simulink model "SEMINAR_DFIG_withsubsys"  (R2014a)
settings: Solver=ode23tb  StartTime=0.0  StopTime=1  FixedStep=1e-9  RelTol=1e-8  AbsTol=1e-8
libraries: powerlib x18, powerlib_meascontrol x13, simulink x7
settings Model: BufferReuse=off  Creator=user  LastModifiedBy=ninad gaikawad
settings SolverCC: MaxConsecutiveZCs=1000000  MaxConsecutiveMinStep=1000000  ZeroCrossAlgorithm=Adaptive  SolverResetMethod=Robust
settings OptimizationCC: BlockReduction=off  OptimizeBlockIOStorage=off  BufferReuse=off  GlobalBufferReuse=off  ExpressionFolding=off  LocalBlockOutputs=off

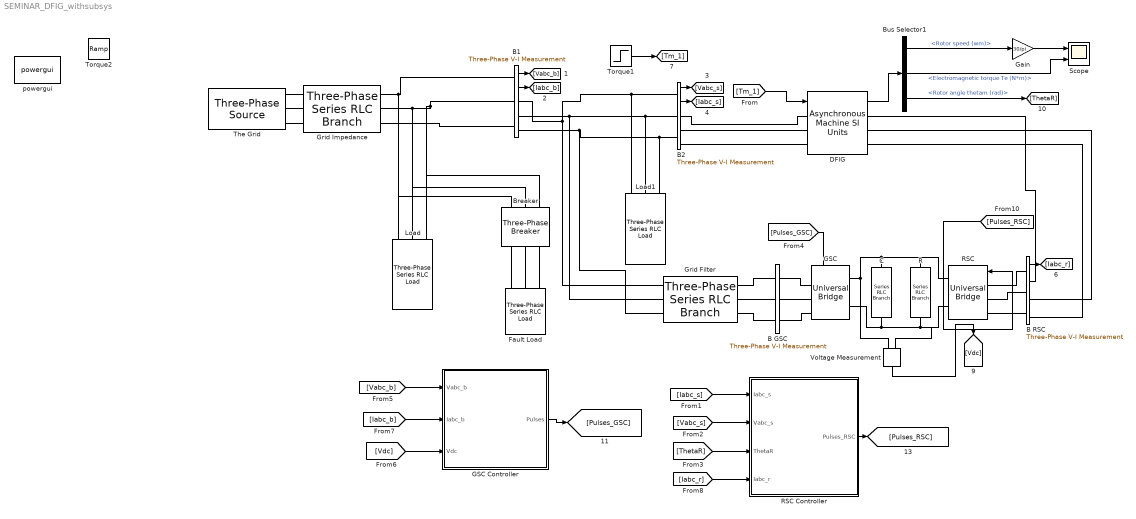
== system SEMINAR_DFIG_withsubsys ==
  B GSC : powerlib/Measurements/Three-Phase V-I Measurement  VoltageMeasurement=no  SetLabelV=off  LabelV=Vabc  Vpu=off  VpuLL=off  CurrentMeasurement=no  SetLabelI=off  LabelI=Iabc  Ipu=off  Pbase=100e6  Vbase=500e3  OutputType=Complex  PhasorSimulation=off  PSBequivalent=0
  B RSC : powerlib/Measurements/Three-Phase V-I Measurement  VoltageMeasurement=no  SetLabelV=off  LabelV=Vabc  Vpu=off  VpuLL=off  CurrentMeasurement=yes  SetLabelI=off  LabelI=Iabc  Ipu=off  Pbase=100e6  Vbase=500e3  OutputType=Complex  PhasorSimulation=off  PSBequivalent=0
  B1 : powerlib/Measurements/Three-Phase V-I Measurement  VoltageMeasurement=phase-to-ground  SetLabelV=off  LabelV=Vabc  Vpu=off  VpuLL=off  CurrentMeasurement=yes  SetLabelI=off  LabelI=Iabc  Ipu=off  Pbase=100e6  Vbase=500e3  OutputType=Complex  PhasorSimulation=off  PSBequivalent=0
  B2 : powerlib/Measurements/Three-Phase V-I Measurement  VoltageMeasurement=phase-to-ground  SetLabelV=off  LabelV=Vabc  Vpu=off  VpuLL=off  CurrentMeasurement=yes  SetLabelI=off  LabelI=Iabc  Ipu=off  Pbase=100e6  Vbase=500e3  OutputType=Complex  PhasorSimulation=off  PSBequivalent=0
  Breaker : powerlib/Elements/Three-Phase Breaker  InitialState=open  SwitchA=on  SwitchB=on  SwitchC=on  SwitchTimes="[1/60  5/60]"  External=off  BreakerResistance=0.01  SnubberResistance=1e6  SnubberCapacitance=inf  Measurements=None
  Bus Selector1 : BusSelector  OutputSignals=Mechanical.Rotor speed (wm),Mechanical.Electromagnetic torque Te (N*m),Mechanical.Rotor angle thetam (rad)
  C : powerlib/Elements/Series RLC Branch  LConnTagsString=__new0  RConnTagsString=__new0  BranchType=C  Resistance=1  Inductance=1e-3  SetiL0=off  InitialCurrent=0  Capacitance=0.0024  Setx0=off  InitialVoltage=0  Measurements=None
  DFIG : powerlib/Machines/Asynchronous Machine SI Units  PresetModel=No  MechanicalLoad=Torque Tm  ShowDetailedParameters=on  RotorType=Wound  ReferenceFrame=Rotor  Units=SI  MeasurementBus=off  NominalParameters=[7.5e3 415 50]  Stator=[1.06 0.2065]  Rotor=[0.80 0.0810]  Cage1=[ 0.022 0.226/377]  Cage2=[ 0.022 0.226/377]  Lm=0.02135  Mechanical=[0.03 0.02187 3]  PolePairs=2  InitialConditions=[1 0 0 0 0 0 0 0]  SimulateSaturation=off  Saturation=[14.03593122, 27.81365428, 53.79336849, 72.68890987, 97.98006896, 148.6815601, 215.7428561, 302.9841135, 420.4778367 ; 230, 322, 414, 460, 506, 552, 598, 644, 690]  LoadFlowParameters=1492000  TsPowergui=0  TsBlock=-1  IterativeModel=Trapezoidal non iterative  Pmec=0
  Fault Load : powerlib/Elements/Three-Phase Series RLC Load  LConnTagsString=A|B|C  Configuration=Y (grounded)  NominalVoltage=1000  NominalFrequency=60  ActivePower=0.05e+3  InductivePower=0  CapacitivePower=0  Measurements=None  LoadType=constant Z
  GSC : powerlib/Power Electronics/Universal Bridge  Arms=3  SnubberResistance=1e5  SnubberCapacitance=inf  Device=IGBT / Diodes  Ron=1e-3  Lon=0  ForwardVoltages="[  0  0  ]"  ForwardVoltage=0  GTOparameters=[ 10e-6 , 20e-6 ]  IGBTparameters=[ 1e-6 , 2e-6 ]  Measurements=None  Measurements_2=None  converterType=Rectifier
  GSC Controller : Subsystem
  Gain : Gain  Gain=30/pi
  Grid Filter : powerlib/Elements/Three-Phase Series RLC Branch  LConnTagsString=A|B|C  RConnTagsString=A|B|C  BranchType=RL  Resistance=0.1  Inductance=0.012  Capacitance=1e-6  Measurements=None
  Grid Impedance : powerlib/Elements/Three-Phase Series RLC Branch  LConnTagsString=A|B|C  RConnTagsString=A|B|C  BranchType=RL  Resistance=1  Inductance=1e-3  Capacitance=1e-6  Measurements=None
  Load : powerlib/Elements/Three-Phase Series RLC Load  LConnTagsString=A|B|C  Configuration=Y (grounded)  NominalVoltage=1000  NominalFrequency=50  ActivePower=5e+3  InductivePower=0  CapacitivePower=0  Measurements=None  LoadType=constant Z
  Load1 : powerlib/Elements/Three-Phase Series RLC Load  LConnTagsString=A|B|C  Configuration=Y (grounded)  NominalVoltage=1000  NominalFrequency=50  ActivePower=5e+4  InductivePower=0  CapacitivePower=0  Measurements=None  LoadType=constant Z
  R : powerlib/Elements/Series RLC Branch  LConnTagsString=__new0  RConnTagsString=__new0  BranchType=R  Resistance=1  Inductance=1e-3  SetiL0=off  InitialCurrent=0  Capacitance=1e-6  Setx0=off  InitialVoltage=0  Measurements=None
  RSC : powerlib/Power Electronics/Universal Bridge  Arms=3  SnubberResistance=1e5  SnubberCapacitance=inf  Device=IGBT / Diodes  Ron=1e-3  Lon=0  ForwardVoltages="[  0  0  ]"  ForwardVoltage=0  GTOparameters=[ 10e-6 , 20e-6 ]  IGBTparameters=[ 1e-6 , 2e-6 ]  Measurements=None  Measurements_2=None  converterType=Rectifier
  RSC Controller : Subsystem
  Scope : Scope  NumInputPorts=2
      settings: YMin=-5~-5  YMax=5~5
  The Grid : powerlib/Electrical Sources/Three-Phase Source  Voltage=415  PhaseAngle=0  Frequency=50  InternalConnection=Yg  SpecifyImpedance=off  Resistance=0.8929  Inductance=0  ShortCircuitLevel=100e6  BaseVoltage=25e3  XRratio=7  BusType=swing  Pref=0  Qref=0  Qmin=-inf  Qmax=inf
  Torque1 : Step  Time=0.5  After=-25  SampleTime=0
  Torque2 : simulink/Sources/Ramp  slope=-1  start=0  X0=0
  Voltage Measurement : powerlib/Measurements/Voltage Measurement  PhasorSimulation=off  OutputType=Complex  PSBequivalent=0
  powergui : powerlib/powergui  Priority=1  SimulationMode=Continuous  SolverType=Tustin  SampleTime=50e-6  frequency=60  SPID=off  DisableSnubberDevices=off  DisableRonSwitches=off  DisableVfSwitches=off  SwTol=0  Interpol=off  DisplayEquations=off  Ts=0  methode=off  frequencyindice=50  Pbase=100e6  ErrMax=1e-4  Iterations=50  UnitsV=kV  UnitsW=MW  FunctionMessages=off  echomessages=off  HookPort=off  EnableUseOfTLC=off  x0status=blocks  RestoreLinks=warning  ResistiveCurrentMeasurement=off  Frange=[0:2:500]  Ylog=off  Xlog=on  ShowGrid=off  save=off  variable=ZData  structure=0  ZoomFFT=off  StartTime=0.0  cycles=1  DisplayStyle=1  fundamental=60  FreqAxis=off  MaxFrequency=1000  frequencyindicesteady=1  RmsSteady=1  display=off
  wires:
  DFIG/1 -> Bus Selector1/1
  B1/1 -> [Vabc_b]
  B1/2 -> [Iabc_b]
  B2/1 -> [Vabc_s]
  B2/2 -> [Iabc_s]
  B RSC/1 -> [Iabc_r]
  Torque1/1 -> [Tm_1]
  [Tm_1] -> DFIG/1
  Voltage Measurement/1 -> [Vdc]
  [Pulses_GSC] -> GSC/1
  [Vabc_b] -> GSC Controller/1(Vabc_b)
  [Vdc] -> GSC Controller/3(Vdc)
  GSC Controller/1(Pulses) -> [Pulses_GSC]
  [Iabc_b] -> GSC Controller/2(Iabc_b)
  Bus Selector1/1 -> Gain/1  "<Rotor speed (wm)>"
  Gain/1 -> Scope/1
  Bus Selector1/3 -> [ThetaR]  "<Rotor angle thetam (rad)>"
  Bus Selector1/2 -> Scope/2  "<Electromagnetic torque Te (N*m)>"
  [Iabc_s] -> RSC Controller/1(Iabc_s)
  [ThetaR] -> RSC Controller/3(ThetaR)
  [Iabc_r] -> RSC Controller/4(Iabc_r)
  RSC Controller/1(Pulses_RSC) -> [Pulses_RSC]
  [Vabc_s] -> RSC Controller/2(Vabc_s)
  [Pulses_RSC] -> RSC/1
  connections:
  GSC/RConn1 -- RSC/RConn1 -- R/LConn1 -- C/LConn1 -- Voltage Measurement/LConn1
  GSC/RConn2 -- Voltage Measurement/LConn2 -- RSC/RConn2 -- R/RConn1 -- C/RConn1
  The Grid/RConn1 -- Grid Impedance/LConn1
  The Grid/RConn2 -- Grid Impedance/LConn2
  The Grid/RConn3 -- Grid Impedance/LConn3
  Breaker/RConn1 -- Fault Load/LConn1
  Breaker/RConn2 -- Fault Load/LConn2
  Grid Impedance/RConn2 -- Breaker/LConn2 -- Load/LConn2 -- Breaker/LConn3 -- Load/LConn3 -- B1/LConn2
  Grid Impedance/RConn3 -- B1/LConn3
  B1/RConn2 -- Grid Filter/LConn2 -- Load1/LConn2 -- B2/LConn2
  B1/RConn3 -- Grid Filter/LConn3 -- Load1/LConn3 -- B2/LConn3
  B2/LConn1 -- Load1/LConn1 -- Grid Filter/LConn1 -- B1/RConn1
  Grid Impedance/RConn1 -- Breaker/LConn1 -- Load/LConn1 -- B1/LConn1
  Fault Load/LConn3 -- Breaker/RConn3
  B2/RConn1 -- DFIG/LConn1
  B2/RConn2 -- DFIG/LConn2
  B2/RConn3 -- DFIG/LConn3
  Grid Filter/RConn1 -- B GSC/LConn1
  Grid Filter/RConn2 -- B GSC/LConn2
  Grid Filter/RConn3 -- B GSC/LConn3
  B GSC/RConn3 -- GSC/LConn3
  B GSC/RConn2 -- GSC/LConn2
  B GSC/RConn1 -- GSC/LConn1
  RSC/LConn1 -- B RSC/LConn1
  RSC/LConn2 -- B RSC/LConn2
  RSC/LConn3 -- B RSC/LConn3
  DFIG/RConn1 -- B RSC/RConn1
  DFIG/RConn2 -- B RSC/RConn2
  DFIG/RConn3 -- B RSC/RConn3

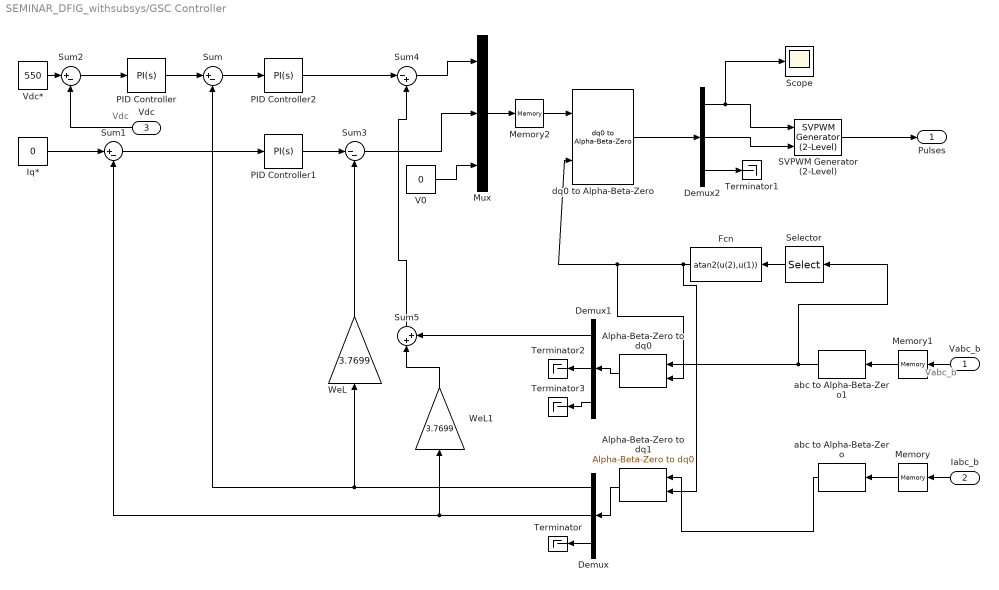
== system SEMINAR_DFIG_withsubsys/GSC Controller ==
  note: Vdc
  note: Vabc_b
  Vabc_b : Inport
  Iabc_b : Inport  Port=2
  Vdc : Inport  Port=3
  Alpha-Beta-Zero to dq0 : powerlib_meascontrol/Transformations/Alpha-Beta-Zero to dq0  Alignment=Aligned with phase A axis
  Alpha-Beta-Zero to dq1 : powerlib_meascontrol/Transformations/Alpha-Beta-Zero to dq0  Alignment=Aligned with phase A axis
  Demux : Demux  Outputs=3
  Demux1 : Demux  Outputs=3
  Demux2 : Demux  Outputs=3
  Fcn : Fcn  Expr=atan2(u(2),u(1))
  Iq* : Constant  Value=0
  Memory : Memory  X0=1
  Memory1 : Memory  X0=100
  Memory2 : Memory  X0=1
  Mux : Mux  Inputs=3
  PID Controller : simulink/Continuous/PID Controller  Controller=PI  TimeDomain=Continuous-time  SampleTime=1  IntegratorMethod=Forward Euler  FilterMethod=Forward Euler  Form=Parallel  P=0.028073571427237  I=0.0618958834223804  D=0  N=100  InitialConditionSource=internal  InitialConditionForIntegrator=0  InitialConditionForFilter=0  ExternalReset=none  LimitOutput=off  UpperSaturationLimit=1  LowerSaturationLimit=-1  LinearizeAsGain=on  AntiWindupMode=none  Kb=1  TrackingMode=off  Kt=1  PParamMin=[]  PParamMax=[]  IParamMin=[]  IParamMax=[]  DParamMin=[]  DParamMax=[]  NParamMin=[]  NParamMax=[]  KbParamMin=[]  KbParamMax=[]  KtParamMin=[]  KtParamMax=[]  POutMin=[]  POutMax=[]  IOutMin=[]  IOutMax=[]  DOutMin=[]  DOutMax=[]  NOutMin=[]  NOutMax=[]  KbOutMin=[]  KbOutMax=[]  KtOutMin=[]  KtOutMax=[]  IntegratorOutMin=[]  IntegratorOutMax=[]  FilterOutMin=[]  FilterOutMax=[]  SumOutMin=[]  SumOutMax=[]  SumI1OutMin=[]  SumI1OutMax=[]  SumI2OutMin=[]  SumI2OutMax=[]  SumI3OutMin=[]  SumI3OutMax=[]  SumDOutMin=[]  SumDOutMax=[]  SaturationOutMin=[]  SaturationOutMax=[]  IntegratorContinuousStateAttributes=''  IntegratorStateMustResolveToSignalObject=off  IntegratorRTWStateStorageClass=Auto  FilterContinuousStateAttributes=''  FilterStateMustResolveToSignalObject=off  FilterRTWStateStorageClass=Auto
  PID Controller1 : simulink/Continuous/PID Controller  Controller=PI  TimeDomain=Continuous-time  SampleTime=1  IntegratorMethod=Forward Euler  FilterMethod=Forward Euler  Form=Parallel  P=8.37826727980584  I=0.0516922409916327  D=0  N=100  InitialConditionSource=internal  InitialConditionForIntegrator=0  InitialConditionForFilter=0  ExternalReset=none  LimitOutput=off  UpperSaturationLimit=1  LowerSaturationLimit=-1  LinearizeAsGain=on  AntiWindupMode=none  Kb=1  TrackingMode=off  Kt=1  PParamMin=[]  PParamMax=[]  IParamMin=[]  IParamMax=[]  DParamMin=[]  DParamMax=[]  NParamMin=[]  NParamMax=[]  KbParamMin=[]  KbParamMax=[]  KtParamMin=[]  KtParamMax=[]  POutMin=[]  POutMax=[]  IOutMin=[]  IOutMax=[]  DOutMin=[]  DOutMax=[]  NOutMin=[]  NOutMax=[]  KbOutMin=[]  KbOutMax=[]  KtOutMin=[]  KtOutMax=[]  IntegratorOutMin=[]  IntegratorOutMax=[]  FilterOutMin=[]  FilterOutMax=[]  SumOutMin=[]  SumOutMax=[]  SumI1OutMin=[]  SumI1OutMax=[]  SumI2OutMin=[]  SumI2OutMax=[]  SumI3OutMin=[]  SumI3OutMax=[]  SumDOutMin=[]  SumDOutMax=[]  SaturationOutMin=[]  SaturationOutMax=[]  IntegratorContinuousStateAttributes=''  IntegratorStateMustResolveToSignalObject=off  IntegratorRTWStateStorageClass=Auto  FilterContinuousStateAttributes=''  FilterStateMustResolveToSignalObject=off  FilterRTWStateStorageClass=Auto
  PID Controller2 : simulink/Continuous/PID Controller  Controller=PI  TimeDomain=Continuous-time  SampleTime=1  IntegratorMethod=Forward Euler  FilterMethod=Forward Euler  Form=Parallel  P=8.37826727980584  I=0.0516922409916327  D=0  N=100  InitialConditionSource=internal  InitialConditionForIntegrator=0  InitialConditionForFilter=0  ExternalReset=none  LimitOutput=off  UpperSaturationLimit=1  LowerSaturationLimit=-1  LinearizeAsGain=on  AntiWindupMode=none  Kb=1  TrackingMode=off  Kt=1  PParamMin=[]  PParamMax=[]  IParamMin=[]  IParamMax=[]  DParamMin=[]  DParamMax=[]  NParamMin=[]  NParamMax=[]  KbParamMin=[]  KbParamMax=[]  KtParamMin=[]  KtParamMax=[]  POutMin=[]  POutMax=[]  IOutMin=[]  IOutMax=[]  DOutMin=[]  DOutMax=[]  NOutMin=[]  NOutMax=[]  KbOutMin=[]  KbOutMax=[]  KtOutMin=[]  KtOutMax=[]  IntegratorOutMin=[]  IntegratorOutMax=[]  FilterOutMin=[]  FilterOutMax=[]  SumOutMin=[]  SumOutMax=[]  SumI1OutMin=[]  SumI1OutMax=[]  SumI2OutMin=[]  SumI2OutMax=[]  SumI3OutMin=[]  SumI3OutMax=[]  SumDOutMin=[]  SumDOutMax=[]  SaturationOutMin=[]  SaturationOutMax=[]  IntegratorContinuousStateAttributes=''  IntegratorStateMustResolveToSignalObject=off  IntegratorRTWStateStorageClass=Auto  FilterContinuousStateAttributes=''  FilterStateMustResolveToSignalObject=off  FilterRTWStateStorageClass=Auto
  SVPWM Generator (2-Level) : powerlib_meascontrol/Pulse & Signal Generators/SVPWM Generator (2-Level)  InputType=alpha-beta components  SwitchingPattern=Pattern #1  Fc=27*50  ParUref=[0.8 -30 50]  Ts=0
  Scope : Scope
  Selector : Selector  InputPortWidth=3  Indices=[1 2]
  Sum : Sum  Inputs=|+-
  Sum1 : Sum  Inputs=|+-
  Sum2 : Sum  Inputs=|+-
  Sum3 : Sum  Inputs=|--
  Sum4 : Sum  Inputs=|-+
  Sum5 : Sum  Inputs=|++
  Terminator{,1..3} (4 alike) : Terminator
  V0 : Constant  Value=0
  Vdc* : Constant  Value=550
  WeL : Gain  Gain=3.7699
  WeL1 : Gain  Gain=3.7699
  abc to Alpha-Beta-Zero : powerlib_meascontrol/Transformations/abc to Alpha-Beta-Zero
  abc to Alpha-Beta-Zero1 : powerlib_meascontrol/Transformations/abc to Alpha-Beta-Zero
  dq0 to Alpha-Beta-Zero : powerlib_meascontrol/Transformations/dq0 to Alpha-Beta-Zero  Alignment=90 degrees behind phase A axis
  Pulses : Outport
  wires:
  Demux1/3 -> Terminator3/1
  Demux/3 -> Terminator/1
  Alpha-Beta-Zero to dq1/1 -> Demux/1
  Fcn/1 -> Alpha-Beta-Zero to dq1/2, dq0 to Alpha-Beta-Zero/2, Alpha-Beta-Zero to dq0/2
  abc to Alpha-Beta-Zero1/1 -> Selector/1, Alpha-Beta-Zero to dq0/1
  abc to Alpha-Beta-Zero/1 -> Alpha-Beta-Zero to dq1/1
  Alpha-Beta-Zero to dq0/1 -> Demux1/1
  Vabc_b/1 -> Memory1/1
  Demux1/2 -> Terminator2/1
  Iabc_b/1 -> Memory/1
  Selector/1 -> Fcn/1
  Demux2/3 -> Terminator1/1
  Demux2/2 -> SVPWM Generator (2-Level)/2
  Demux2/1 -> Scope/1, SVPWM Generator (2-Level)/1
  dq0 to Alpha-Beta-Zero/1 -> Demux2/1
  SVPWM Generator (2-Level)/1 -> Pulses/1
  Mux/1 -> Memory2/1
  Sum4/1 -> Mux/1
  PID Controller1/1 -> Sum3/1
  Demux/1 -> Sum/2, WeL/1
  Demux1/1 -> Sum5/2
  PID Controller2/1 -> Sum4/1
  Demux/2 -> Sum1/2, WeL1/1
  Sum1/1 -> PID Controller1/1
  Sum5/1 -> Sum4/2
  Sum3/1 -> Mux/2
  WeL1/1 -> Sum5/1
  PID Controller/1 -> Sum/1
  Iq*/1 -> Sum1/1
  WeL/1 -> Sum3/2
  Sum2/1 -> PID Controller/1
  Vdc*/1 -> Sum2/1
  V0/1 -> Mux/3
  Sum/1 -> PID Controller2/1
  Vdc/1 -> Sum2/2
  Memory1/1 -> abc to Alpha-Beta-Zero1/1
  Memory/1 -> abc to Alpha-Beta-Zero/1
  Memory2/1 -> dq0 to Alpha-Beta-Zero/1

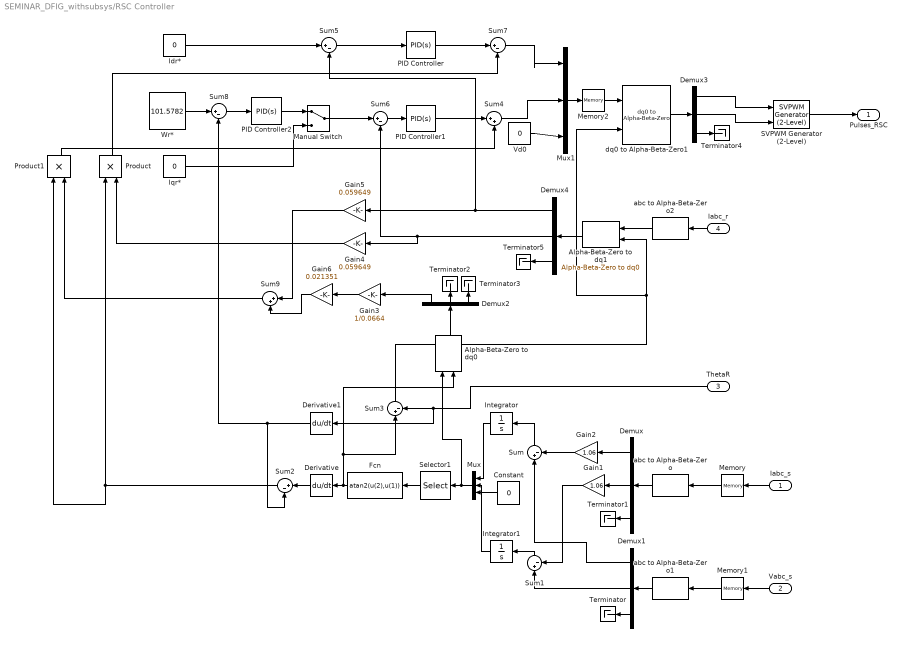
== system SEMINAR_DFIG_withsubsys/RSC Controller ==
  Iabc_s : Inport
  Vabc_s : Inport  Port=2
  ThetaR : Inport  Port=3
  Iabc_r : Inport  Port=4
  Alpha-Beta-Zero to dq0 : powerlib_meascontrol/Transformations/Alpha-Beta-Zero to dq0  Alignment=90 degrees behind phase A axis
  Alpha-Beta-Zero to dq1 : powerlib_meascontrol/Transformations/Alpha-Beta-Zero to dq0  Alignment=90 degrees behind phase A axis
  Constant : Constant  Value=0
  Demux{,1..4} (5 alike) : Demux  Outputs=3
  Derivative : Derivative
  Derivative1 : Derivative
  Fcn : Fcn  Expr=atan2(u(2),u(1))
  Gain1 : Gain  Gain=1.06
  Gain2 : Gain  Gain=1.06
  Gain3 : Gain  Gain=1/0.0664
  Gain4 : Gain  Gain=0.059649
  Gain5 : Gain  Gain=0.059649
  Gain6 : Gain  Gain=0.021351
  Idr* : Constant  Value=0
  Integrator : Integrator
  Integrator1 : Integrator
  Iqr* : Constant  Value=0
  Manual Switch : ManualSwitch
  Memory : Memory  X0=1
  Memory1 : Memory  X0=100
  Memory2 : Memory  X0=1
  Mux : Mux  Inputs=3
  Mux1 : Mux  Inputs=3
  PID Controller : simulink/Continuous/PID Controller  Controller=PID  TimeDomain=Continuous-time  SampleTime=1  IntegratorMethod=Forward Euler  FilterMethod=Forward Euler  Form=Parallel  P=8.37133654779394  I=0.0658637916646154  D=0  N=100  InitialConditionSource=internal  InitialConditionForIntegrator=0  InitialConditionForFilter=0  ExternalReset=none  LimitOutput=off  UpperSaturationLimit=inf  LowerSaturationLimit=-inf  LinearizeAsGain=on  AntiWindupMode=none  Kb=1  TrackingMode=off  Kt=1  PParamMin=[]  PParamMax=[]  IParamMin=[]  IParamMax=[]  DParamMin=[]  DParamMax=[]  NParamMin=[]  NParamMax=[]  KbParamMin=[]  KbParamMax=[]  KtParamMin=[]  KtParamMax=[]  POutMin=[]  POutMax=[]  IOutMin=[]  IOutMax=[]  DOutMin=[]  DOutMax=[]  NOutMin=[]  NOutMax=[]  KbOutMin=[]  KbOutMax=[]  KtOutMin=[]  KtOutMax=[]  IntegratorOutMin=[]  IntegratorOutMax=[]  FilterOutMin=[]  FilterOutMax=[]  SumOutMin=[]  SumOutMax=[]  SumI1OutMin=[]  SumI1OutMax=[]  SumI2OutMin=[]  SumI2OutMax=[]  SumI3OutMin=[]  SumI3OutMax=[]  SumDOutMin=[]  SumDOutMax=[]  SaturationOutMin=[]  SaturationOutMax=[]  IntegratorContinuousStateAttributes=''  IntegratorStateMustResolveToSignalObject=off  IntegratorRTWStateStorageClass=Auto  FilterContinuousStateAttributes=''  FilterStateMustResolveToSignalObject=off  FilterRTWStateStorageClass=Auto
  PID Controller1 : simulink/Continuous/PID Controller  Controller=PID  TimeDomain=Continuous-time  SampleTime=1  IntegratorMethod=Forward Euler  FilterMethod=Forward Euler  Form=Parallel  P=8.37133654779394  I=0.0658637916646154  D=0  N=100  InitialConditionSource=internal  InitialConditionForIntegrator=0  InitialConditionForFilter=0  ExternalReset=none  LimitOutput=off  UpperSaturationLimit=inf  LowerSaturationLimit=-inf  LinearizeAsGain=on  AntiWindupMode=none  Kb=1  TrackingMode=off  Kt=1  PParamMin=[]  PParamMax=[]  IParamMin=[]  IParamMax=[]  DParamMin=[]  DParamMax=[]  NParamMin=[]  NParamMax=[]  KbParamMin=[]  KbParamMax=[]  KtParamMin=[]  KtParamMax=[]  POutMin=[]  POutMax=[]  IOutMin=[]  IOutMax=[]  DOutMin=[]  DOutMax=[]  NOutMin=[]  NOutMax=[]  KbOutMin=[]  KbOutMax=[]  KtOutMin=[]  KtOutMax=[]  IntegratorOutMin=[]  IntegratorOutMax=[]  FilterOutMin=[]  FilterOutMax=[]  SumOutMin=[]  SumOutMax=[]  SumI1OutMin=[]  SumI1OutMax=[]  SumI2OutMin=[]  SumI2OutMax=[]  SumI3OutMin=[]  SumI3OutMax=[]  SumDOutMin=[]  SumDOutMax=[]  SaturationOutMin=[]  SaturationOutMax=[]  IntegratorContinuousStateAttributes=''  IntegratorStateMustResolveToSignalObject=off  IntegratorRTWStateStorageClass=Auto  FilterContinuousStateAttributes=''  FilterStateMustResolveToSignalObject=off  FilterRTWStateStorageClass=Auto
  PID Controller2 : simulink/Continuous/PID Controller  Controller=PID  TimeDomain=Continuous-time  SampleTime=1  IntegratorMethod=Forward Euler  FilterMethod=Forward Euler  Form=Parallel  P=35.0827060032723  I=33.1490428648513  D=0  N=100  InitialConditionSource=internal  InitialConditionForIntegrator=0  InitialConditionForFilter=0  ExternalReset=none  LimitOutput=off  UpperSaturationLimit=inf  LowerSaturationLimit=-inf  LinearizeAsGain=on  AntiWindupMode=none  Kb=1  TrackingMode=off  Kt=1  PParamMin=[]  PParamMax=[]  IParamMin=[]  IParamMax=[]  DParamMin=[]  DParamMax=[]  NParamMin=[]  NParamMax=[]  KbParamMin=[]  KbParamMax=[]  KtParamMin=[]  KtParamMax=[]  POutMin=[]  POutMax=[]  IOutMin=[]  IOutMax=[]  DOutMin=[]  DOutMax=[]  NOutMin=[]  NOutMax=[]  KbOutMin=[]  KbOutMax=[]  KtOutMin=[]  KtOutMax=[]  IntegratorOutMin=[]  IntegratorOutMax=[]  FilterOutMin=[]  FilterOutMax=[]  SumOutMin=[]  SumOutMax=[]  SumI1OutMin=[]  SumI1OutMax=[]  SumI2OutMin=[]  SumI2OutMax=[]  SumI3OutMin=[]  SumI3OutMax=[]  SumDOutMin=[]  SumDOutMax=[]  SaturationOutMin=[]  SaturationOutMax=[]  IntegratorContinuousStateAttributes=''  IntegratorStateMustResolveToSignalObject=off  IntegratorRTWStateStorageClass=Auto  FilterContinuousStateAttributes=''  FilterStateMustResolveToSignalObject=off  FilterRTWStateStorageClass=Auto
  Product : Product
  Product1 : Product
  SVPWM Generator (2-Level) : powerlib_meascontrol/Pulse & Signal Generators/SVPWM Generator (2-Level)  InputType=alpha-beta components  SwitchingPattern=Pattern #1  Fc=27*50  ParUref=[0.8 -30 50]  Ts=0
  Selector1 : Selector  InputPortWidth=3  Indices=[1 2]
  Sum{,1..3,5..8} (8 alike) : Sum  Inputs=|+-
  Sum4 : Sum  Inputs=|++
  Sum9 : Sum  Inputs=|++
  Terminator{,1..5} (6 alike) : Terminator
  Vd0 : Constant  Value=0
  Wr* : Constant  Value=101.5782
  abc to Alpha-Beta-Zero : powerlib_meascontrol/Transformations/abc to Alpha-Beta-Zero
  abc to Alpha-Beta-Zero1 : powerlib_meascontrol/Transformations/abc to Alpha-Beta-Zero
  abc to Alpha-Beta-Zero2 : powerlib_meascontrol/Transformations/abc to Alpha-Beta-Zero
  dq0 to Alpha-Beta-Zero1 : powerlib_meascontrol/Transformations/dq0 to Alpha-Beta-Zero  Alignment=90 degrees behind phase A axis
  Pulses_RSC : Outport
  wires:
  Gain2/1 -> Sum/2
  Sum/1 -> Integrator/1
  Demux/2 -> Gain1/1
  Demux1/2 -> Sum1/1
  Demux/1 -> Gain2/1
  Demux1/1 -> Sum/1
  SVPWM Generator (2-Level)/1 -> Pulses_RSC/1
  dq0 to Alpha-Beta-Zero1/1 -> Demux3/1
  Demux3/1 -> SVPWM Generator (2-Level)/1
  Demux3/3 -> Terminator4/1
  Demux3/2 -> SVPWM Generator (2-Level)/2
  Vabc_s/1 -> Memory1/1
  Iabc_s/1 -> Memory/1
  Integrator1/1 -> Mux/2
  Constant/1 -> Mux/3
  Selector1/1 -> Fcn/1
  Sum1/1 -> Integrator1/1
  ThetaR/1 -> Derivative1/1, Sum3/2
  Gain4/1 -> Product/2
  Mux/1 -> Alpha-Beta-Zero to dq0/1, Selector1/1
  Gain1/1 -> Sum1/2
  Integrator/1 -> Mux/1
  Fcn/1 -> Sum3/1, Alpha-Beta-Zero to dq0/2, Derivative/1
  Derivative/1 -> Sum2/1
  Sum2/1 -> Product1/1, Product/1
  Demux4/1 -> Sum5/2, Gain5/1
  Demux4/2 -> Gain4/1, Sum6/2
  Demux4/3 -> Terminator5/1
  Sum8/1 -> PID Controller2/1
  Derivative1/1 -> Sum8/2, Sum2/2
  Wr*/1 -> Sum8/1
  Gain3/1 -> Gain6/1
  Alpha-Beta-Zero to dq1/1 -> Demux4/1
  Alpha-Beta-Zero to dq0/1 -> Demux2/1
  Sum3/1 -> dq0 to Alpha-Beta-Zero1/2, Alpha-Beta-Zero to dq1/2
  Product1/1 -> Sum4/2
  abc to Alpha-Beta-Zero2/1 -> Alpha-Beta-Zero to dq1/1
  Mux1/1 -> Memory2/1
  Sum7/1 -> Mux1/1
  Vd0/1 -> Mux1/3
  Demux2/3 -> Terminator3/1
  PID Controller1/1 -> Sum4/1
  Demux2/2 -> Terminator2/1
  Demux2/1 -> Gain3/1
  Iabc_r/1 -> abc to Alpha-Beta-Zero2/1
  Product/1 -> Sum7/2
  Sum4/1 -> Mux1/2
  Idr*/1 -> Sum5/1
  Sum5/1 -> PID Controller/1
  Sum9/1 -> Product1/2
  Iqr*/1 -> Manual Switch/2
  Gain6/1 -> Sum9/2
  Manual Switch/1 -> Sum6/1
  PID Controller/1 -> Sum7/1
  Gain5/1 -> Sum9/1
  abc to Alpha-Beta-Zero1/1 -> Demux1/1
  abc to Alpha-Beta-Zero/1 -> Demux/1
  Sum6/1 -> PID Controller1/1
  PID Controller2/1 -> Manual Switch/1
  Demux/3 -> Terminator1/1
  Demux1/3 -> Terminator/1
  Memory/1 -> abc to Alpha-Beta-Zero/1
  Memory1/1 -> abc to Alpha-Beta-Zero1/1
  Memory2/1 -> dq0 to Alpha-Beta-Zero1/1
